simulink model "close_circuit_test"  (R2021a)
settings: Solver=VariableStepAuto  StartTime=0.0  StopTime=10.0  RelTol=1e-3
libraries: spsRMSLib x2, spsACVoltageSourceLib x1, spsCurrentMeasurementLib x1, spsLinearTransformerLib x1, spsPowerLib x1, spsVoltageMeasurementLib x1, spspowerguiLib x1
settings Model: Creator=LENOVO  LastModifiedBy=LENOVO

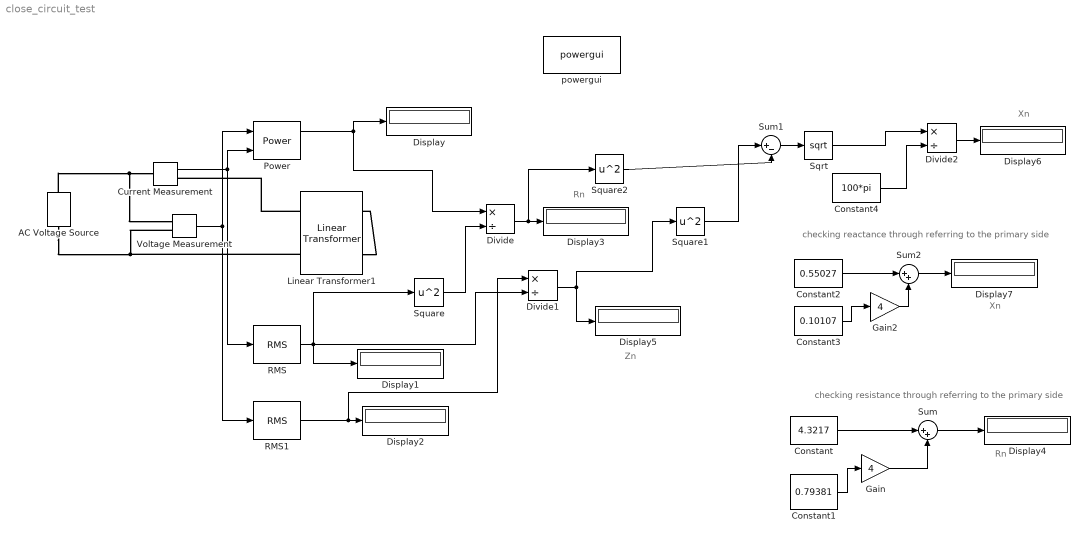
== system close_circuit_test ==
  note: Zn
  note: Rn
  note: Xn
  note: checking resistance through referring to the primary side
  note: Rn
  note: checking reactance through referring to the primary side
  note: Xn
  AC Voltage Source : spsACVoltageSourceLib/AC Voltage Source  Amplitude=220*sqrt(2)  Phase=0  Frequency=50  SampleTime=0  Measurements=None  BusType=swing  Pref=10e3  Qref=0  Qmin=-inf  Qmax=+inf
  Constant : Constant  Value=4.3217
  Constant1 : Constant  Value=0.79381
  Constant2 : Constant  Value=0.55027
  Constant3 : Constant  Value=0.10107
  Constant4 : Constant  Value=100*pi
  Current Measurement : spsCurrentMeasurementLib/Current Measurement  PhasorSimulation=off  OutputType=Complex  PSBequivalent=0
  Display{,1..7} (8 alike) : Display
  Divide : Product  Inputs=*/
  Divide1 : Product  Inputs=*/
  Divide2 : Product  Inputs=*/
  Gain : Gain  Gain=4
  Gain2 : Gain  Gain=4
  Linear Transformer1 : spsLinearTransformerLib/Linear Transformer  UNITS=SI  NominalPower=[ 250e6 50 ]  winding1=[220 4.3217 0.55027]  winding2=[110 0.79381 0.10107]  ThreeWindings=off  winding3=[3.15e+05 0.7938 0.10107]  RmLm=[1.0804e+06 3439.2]  Measurements=None  DataType=on
  Power : spsPowerLib/Power  Freq=50  Vinit=[1, 0]  Iinit=[1, 0]  Ts=0
      settings: SourceProductBaseCode=PS
  RMS : spsRMSLib/RMS  TrueRMS=on  Freq=50  RMSInit=0  Ts=0
  RMS1 : spsRMSLib/RMS  TrueRMS=on  Freq=50  RMSInit=0  Ts=0
  Sqrt : Sqrt  SaturateOnIntegerOverflow=on
  Square : Math  Operator=square  SaturateOnIntegerOverflow=on
  Square1 : Math  Operator=square  SaturateOnIntegerOverflow=on
  Square2 : Math  Operator=square  SaturateOnIntegerOverflow=on
  Sum : Sum  Inputs=|++
  Sum1 : Sum  Inputs=|+-
  Sum2 : Sum  Inputs=|++
  Voltage Measurement : spsVoltageMeasurementLib/Voltage Measurement  PhasorSimulation=off  OutputType=Complex  PSBequivalent=0
  powergui : spspowerguiLib/powergui  Priority=1  SimulationMode=Continuous  SampleTime=50e-2  frequency=60  Iterations=50  frequencyindice=50  Pbase=100e6  ErrMax=1e-4  UnitsV=kV  UnitsW=MW  buscounter=0  FunctionMessages=off  echomessages=off  EnableUseOfTLC=off  CurrentSourceSwitches=off  DisableSnubberDevices=off  DisableRonSwitches=off  DisableVfSwitches=off  DisplayEquations=off  AutomaticDiscreteSolvers=off  SolverType=Tustin/Backward Euler (TBE)  Interpol=off  ExternalGateDelay=off  methode=off  Ts=100  x0status=blocks  SPID=on  SwTol=0  HookPort=off  NonlinearTolerance=1e-4  nMaxIteration=100  ContinueOnMaxIteration=off  RestoreLinks=warning  ResistiveCurrentMeasurement=off  Frange=[0:2:500]  Ylog=off  Xlog=on  ShowGrid=off  save=off  variable=ZData  structure=0  ZoomFFT=off  StartTime=0.0  cycles=1  DisplayStyle=1  fundamental=60  FreqAxis=off  MaxFrequency=1000  frequencyindicesteady=1  RmsSteady=1  display=off
  wires:
  Current Measurement/1 -> RMS/1, Power/2
  Voltage Measurement/1 -> RMS1/1, Power/1
  Power/1 -> Divide/1, Display/1
  RMS1/1 -> Divide1/1, Display2/1
  RMS/1 -> Square/1, Divide1/2, Display1/1
  Square/1 -> Divide/2
  Divide/1 -> Square2/1, Display3/1
  Constant1/1 -> Gain/1
  Constant/1 -> Sum/1
  Gain/1 -> Sum/2
  Sum/1 -> Display4/1
  Divide1/1 -> Square1/1, Display5/1
  Square1/1 -> Sum1/1
  Square2/1 -> Sum1/2
  Sum1/1 -> Sqrt/1
  Constant3/1 -> Gain2/1
  Constant2/1 -> Sum2/1
  Gain2/1 -> Sum2/2
  Sum2/1 -> Display7/1
  Sqrt/1 -> Divide2/1
  Constant4/1 -> Divide2/2
  Divide2/1 -> Display6/1
  connections:
  AC Voltage Source/RConn1 -- Current Measurement/LConn1 -- Voltage Measurement/LConn1
  Linear Transformer1/LConn1 -- Current Measurement/RConn1
  AC Voltage Source/LConn1 -- Linear Transformer1/LConn2 -- Voltage Measurement/LConn2
  Linear Transformer1/RConn2 -- Linear Transformer1/RConn1
